simulink model "testinggrounds"  (R2022b)
settings: Solver=VariableStepAuto  StartTime=0.0  StopTime=5340  RelTol=1e-3
libraries: simulink x1, matrix_library x1
settings Model: Creator=izacu  LastModifiedBy=izacu

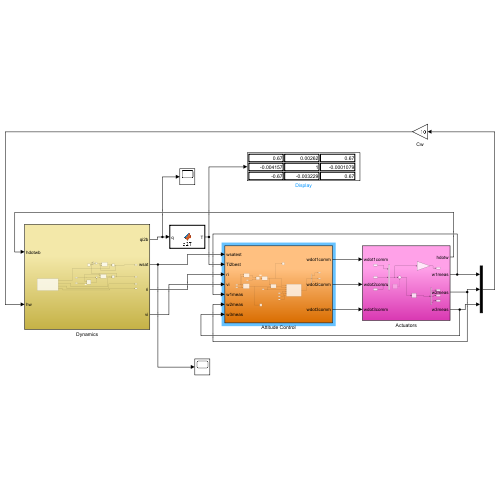
[thumbnail: Simulink's stored preview of the top-level diagram]
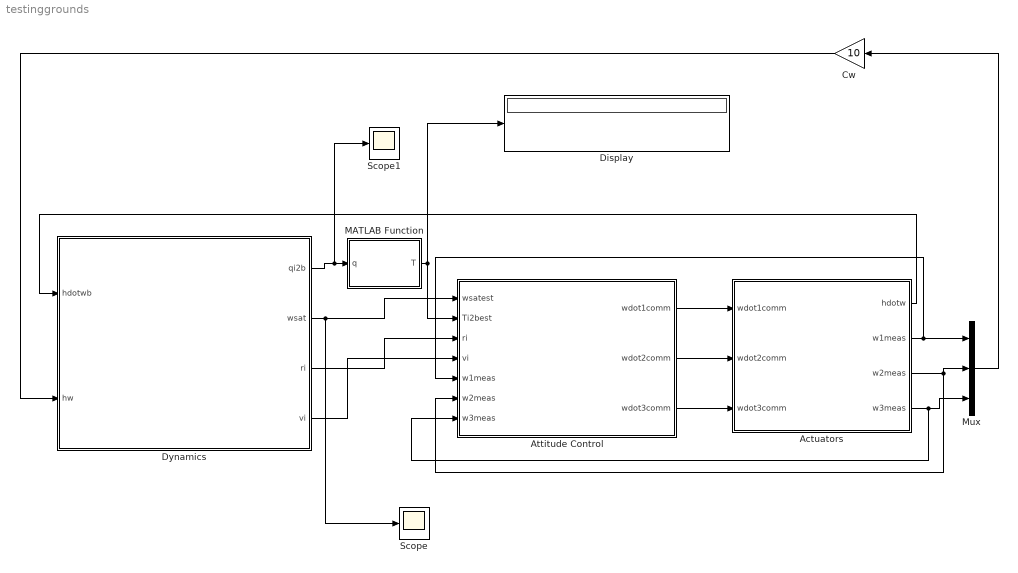
== system testinggrounds ==
  Actuators : Subsystem
  Attitude Control : Subsystem
  Cw : Gain  Gain=10
  Display : Display
  Dynamics : Subsystem
  MATLAB Function : MATLAB Function  TreatAsAtomicUnit=on
  Mux : Mux  Inputs=3
  Scope : Scope
  Scope1 : Scope
  wires:
  Attitude Control/1(wdot1comm) -> Actuators/1(wdot1comm)
  Attitude Control/2(wdot2comm) -> Actuators/2(wdot2comm)
  Attitude Control/3(wdot3comm) -> Actuators/3(wdot3comm)
  Actuators/1(hdotw) -> Dynamics/1(hdotwb)
  Actuators/2(w1meas) -> Attitude Control/5(w1meas), Mux/1
  Actuators/4(w3meas) -> Attitude Control/7(w3meas), Mux/3
  Actuators/3(w2meas) -> Mux/2, Attitude Control/6(w2meas)
  Mux/1 -> Cw/1
  Cw/1 -> Dynamics/2(hw)
  Dynamics/2(wsat) -> Scope/1, Attitude Control/1(wsatest)
  Dynamics/3(ri) -> Attitude Control/3(ri)
  Dynamics/4(vi) -> Attitude Control/4(vi)
  Dynamics/1(qi2b) -> Scope1/1, MATLAB Function/1(q)
  MATLAB Function/1(T) -> Attitude Control/2(Ti2best), Display/1

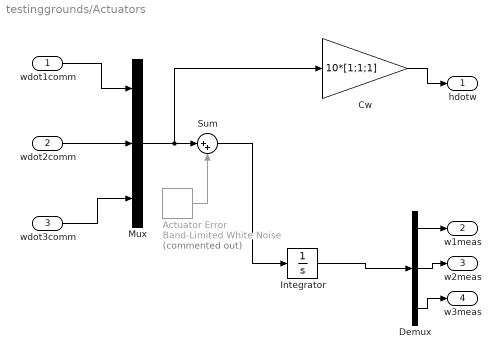
== system testinggrounds/Actuators ==
  wdot1comm : Inport
  wdot2comm : Inport  Port=2
  wdot3comm : Inport  Port=3
  Actuator Error : simulink/Sources/Band-Limited White Noise  Commented=on  Cov=1e-5 * [1;1;1]  Ts=0.1  seed=[23341]
  Cw : Gain  Gain=10*[1;1;1]
  Demux : Demux  Outputs=3
  Integrator : Integrator  InitialCondition=[0;0;0]
  Mux : Mux  Inputs=3
  Sum : Sum  Inputs=|++
  hdotw : Outport
  w1meas : Outport  Port=2
  w2meas : Outport  Port=3
  w3meas : Outport  Port=4
  wires:
  Cw/1 -> hdotw/1
  Demux/3 -> w3meas/1
  Demux/2 -> w2meas/1
  Demux/1 -> w1meas/1
  Integrator/1 -> Demux/1
  Sum/1 -> Integrator/1
  Actuator Error/1 -> Sum/2
  Mux/1 -> Sum/1, Cw/1
  wdot3comm/1 -> Mux/3
  wdot2comm/1 -> Mux/2
  wdot1comm/1 -> Mux/1

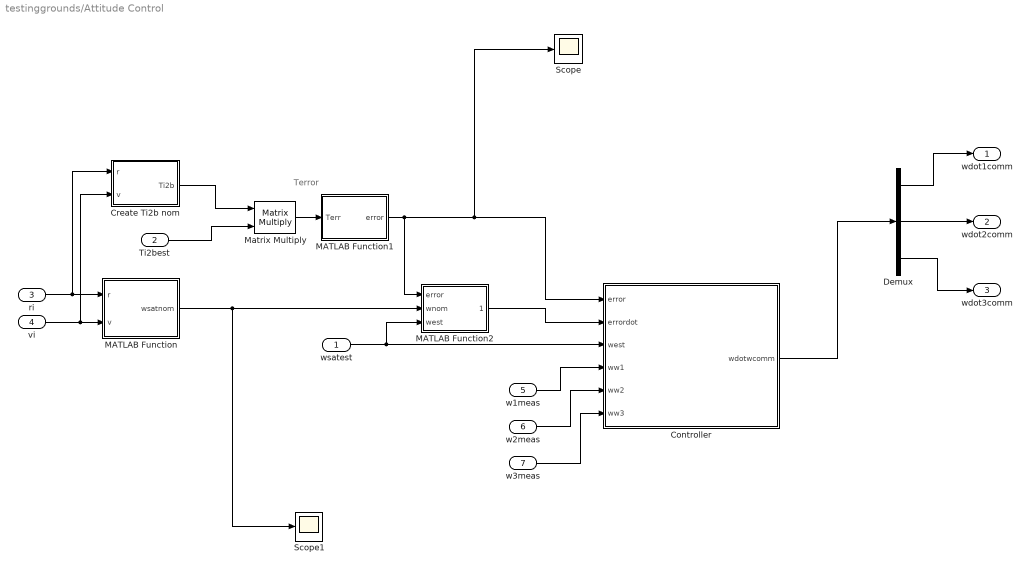
== system testinggrounds/Attitude Control ==
  note: Terror
  wsatest : Inport
  Ti2best : Inport  Port=2
  ri : Inport  Port=3
  vi : Inport  Port=4
  w1meas : Inport  Port=5
  w2meas : Inport  Port=6
  w3meas : Inport  Port=7
  Controller : MATLAB Function  TreatAsAtomicUnit=on
  Create Ti2b nom : MATLAB Function  TreatAsAtomicUnit=on
  Demux : Demux  Outputs=3
  MATLAB Function : MATLAB Function  TreatAsAtomicUnit=on
  MATLAB Function1 : MATLAB Function  TreatAsAtomicUnit=on
  MATLAB Function2 : MATLAB Function  TreatAsAtomicUnit=on
  Matrix Multiply : Product  Multiplication=Matrix(*)
  Scope : Scope
  Scope1 : Scope
  wdot1comm : Outport
  wdot2comm : Outport  Port=2
  wdot3comm : Outport  Port=3
  wires:
  MATLAB Function2/1(errordot) -> Controller/2(errordot)
  w3meas/1 -> Controller/6(ww3)
  w2meas/1 -> Controller/5(ww2)
  w1meas/1 -> Controller/4(ww1)
  wsatest/1 -> MATLAB Function2/3(west), Controller/3(west)
  MATLAB Function/1(wsatnom) -> Scope1/1, MATLAB Function2/2(wnom)
  MATLAB Function1/1(error) -> MATLAB Function2/1(error), Scope/1, Controller/1(error)
  Matrix Multiply/1 -> MATLAB Function1/1(Terr)
  vi/1 -> MATLAB Function/2(v), Create Ti2b nom/2(v)
  ri/1 -> MATLAB Function/1(r), Create Ti2b nom/1(r)
  Demux/3 -> wdot3comm/1
  Demux/2 -> wdot2comm/1
  Demux/1 -> wdot1comm/1
  Ti2best/1 -> Matrix Multiply/2
  Create Ti2b nom/1(Ti2b) -> Matrix Multiply/1
  Controller/1(wdotwcomm) -> Demux/1

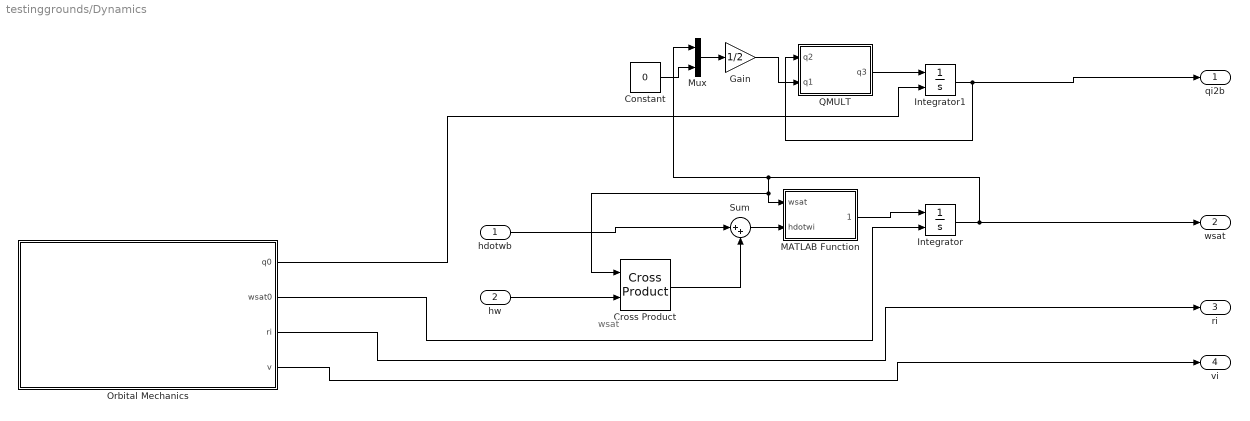
== system testinggrounds/Dynamics ==
  note: wsat
  hdotwb : Inport
  hw : Inport  Port=2
  Constant : Constant  Value=0
  Cross Product : matrix_library/Cross Product
  Gain : Gain  Gain=1/2
  Integrator : Integrator  InitialConditionSource=external
  Integrator1 : Integrator  InitialConditionSource=external
  MATLAB Function : MATLAB Function  TreatAsAtomicUnit=on
  Mux : Mux  Inputs=2
  Orbital Mechanics : Subsystem
  QMULT : MATLAB Function  TreatAsAtomicUnit=on
  Sum : Sum  Inputs=|++
  qi2b : Outport
  wsat : Outport  Port=2
  ri : Outport  Port=3
  vi : Outport  Port=4
  wires:
  Orbital Mechanics/1(q0) -> Integrator1/2
  Constant/1 -> Mux/2
  Mux/1 -> Gain/1
  QMULT/1(q3) -> Integrator1/1
  Integrator1/1 -> QMULT/1(q2), qi2b/1
  Orbital Mechanics/2(wsat0) -> Integrator/2
  Orbital Mechanics/4(v) -> vi/1
  Orbital Mechanics/3(ri) -> ri/1
  Integrator/1 -> Cross Product/1, MATLAB Function/1(wsat), Mux/1, wsat/1
  MATLAB Function/1(wdotsat) -> Integrator/1
  Sum/1 -> MATLAB Function/2(hdotwi)
  Cross Product/1 -> Sum/2
  hdotwb/1 -> Sum/1
  hw/1 -> Cross Product/2
  Gain/1 -> QMULT/2(q1)

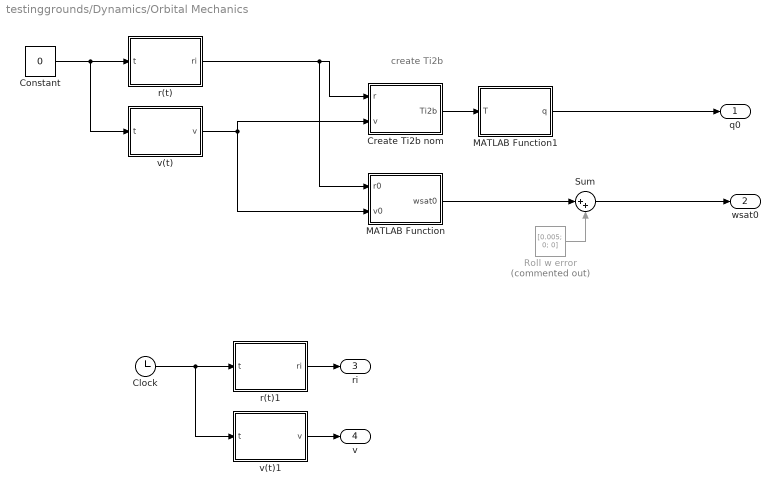
== system testinggrounds/Dynamics/Orbital Mechanics ==
  note: create Ti2b
  Clock : Clock
  Constant : Constant  Value=0
  Create Ti2b nom : MATLAB Function  TreatAsAtomicUnit=on
  MATLAB Function : MATLAB Function  TreatAsAtomicUnit=on
  MATLAB Function1 : MATLAB Function  TreatAsAtomicUnit=on
  Roll w error : Constant  Commented=on  Value=[0.005; 0; 0]
  Sum : Sum  Inputs=|++
  r(t) : MATLAB Function  TreatAsAtomicUnit=on
  r(t)1 : MATLAB Function  TreatAsAtomicUnit=on
  v(t) : MATLAB Function  TreatAsAtomicUnit=on
  v(t)1 : MATLAB Function  TreatAsAtomicUnit=on
  q0 : Outport
  wsat0 : Outport  Port=2
  ri : Outport  Port=3
  v : Outport  Port=4
  wires:
  v(t)1/1(v) -> v/1
  r(t)1/1(ri) -> ri/1
  Clock/1 -> r(t)1/1(t), v(t)1/1(t)
  MATLAB Function1/1(q) -> q0/1
  Create Ti2b nom/1(Ti2b) -> MATLAB Function1/1(T)
  Sum/1 -> wsat0/1
  MATLAB Function/1(wsat0) -> Sum/1
  Roll w error/1 -> Sum/2
  r(t)/1(ri) -> Create Ti2b nom/1(r), MATLAB Function/1(r0)
  v(t)/1(v) -> Create Ti2b nom/2(v), MATLAB Function/2(v0)
  Constant/1 -> r(t)/1(t), v(t)/1(t)

== matlab function testinggrounds/Attitude Control/Controller ==
  data: error input; wdotwcomm output; errordot input; west input; ww1 input; ww2 input; ww3 input
function wdotwcomm = fcn(error,errordot,west,ww1,ww2,ww3)
Jsat = [1000 0 0; 0 500 0; 0 0 600];
Kd = 0.05*eye(3);
Kp = 0.08*eye(3);
Cw = 10;
wdotwcomm = (Jsat*Kd ./ Cw) * error + (Jsat*Kp ./ Cw) * errordot - cross(west, [ww1; ww2; ww3]);

== matlab function testinggrounds/Dynamics/Orbital Mechanics/r(t)1 ==
  data: t input; ri output
function ri = fcn(t)

p = 6.6e6;
mu = 3.986e14;
w = sqrt(mu / (p^3));

ri = (p/sqrt(2)) * [-cos(w*t); sqrt(2)*sin(w*t); cos(w*t)];

== matlab function testinggrounds/Dynamics/MATLAB Function ==
  data: wsat input; wdotsat output; hdotwi input
function wdotsat = fcn(wsat,hdotwi)

J = [1000 0 0;
     0 500 0;
     0 0 600];

wdotsat = inv(J) * (cross(-wsat,(J*wsat)) - hdotwi); %#ok<MINV> 
end

== matlab function testinggrounds/Dynamics/Orbital Mechanics/v(t)1 ==
  data: t input; v output
function v = fcn(t)

p = 6.6e6;
mu = 3.986e14;
w = sqrt(mu / (p^3));

v = (w*p/sqrt(2)) * [sin(w*t); sqrt(2)*cos(w*t); -sin(w*t)];

== matlab function testinggrounds/Dynamics/Orbital Mechanics/r(t) ==
  data: t input; ri output
function ri = fcn(t)

p = 6.6e6;
mu = 3.986e14;
w = sqrt(mu / (p^3));

ri = (p/sqrt(2)) * [-cos(w*t); sqrt(2)*sin(w*t); cos(w*t)];

== matlab function testinggrounds/Dynamics/Orbital Mechanics/v(t) ==
  data: t input; v output
function v = fcn(t)

p = 6.6e6;
mu = 3.986e14;
w = sqrt(mu / (p^3));

v = (w*p/sqrt(2)) * [sin(w*t); sqrt(2)*cos(w*t); -sin(w*t)];

== matlab function testinggrounds/MATLAB Function ==
  data: q input; T output
function T = q2T(q)

T = eye(3) - 2*q(4)*skewsym(q(1:3)) + 2*(skewsym(q(1:3))*skewsym(q(1:3)));

end

function skewed = skewsym(v)
skewed = [0 -v(3) v(2);
          v(3) 0 -v(1);
          -v(2) v(1) 0];
end

== matlab function testinggrounds/Dynamics/QMULT ==
  data: q2 input; q3 output; q1 input
function q3 = qmult(q2,q1)

q3 = [q2(4).*q1(1:3) + q1(4).*q2(1:3) - cross(q2(1:3),q1(1:3));
    q2(4)*q1(4) - dot(q2(1:3),q1(1:3))];

end

== matlab function testinggrounds/Dynamics/Orbital Mechanics/Create Ti2b nom ==
  data: r input; Ti2b output; v input
function Ti2b = fcn(r,v)

xib = -r / norm(r);
yib = v / norm(v);
zib = cross(xib,yib);

Ti2b = [xib'; yib'; zib'];

== matlab function testinggrounds/Dynamics/Orbital Mechanics/MATLAB Function ==
  data: r0 input; wsat0 output; v0 input
function wsat0= fcn(r0,v0)
mu = 3.986e14;
rho = 6.6e6;
wmag = sqrt(mu / rho^3);

h_orbit = cross(r0,v0); % this is the axis our satellite is orbiting about
axis = h_orbit / norm(h_orbit);

wsat0 = wmag .* [0;0;1];

== matlab function testinggrounds/Dynamics/Orbital Mechanics/MATLAB Function1 ==
  data: T input; q output
function q = T2q(T)

q = zeros(4,1);

q(4) = sqrt(.25*(1 + T(1,1) + T(2,2) + T(3,3)));

q = (1/(4*q(4))) .* [T(2,3) - T(3,2); T(3,1) + T(1,3); T(1,2) + T(2,1); 4 * q(4)^2 ];

end

== matlab function testinggrounds/Attitude Control/Create Ti2b nom ==
  data: r input; Ti2b output; v input
function Ti2b = fcn(r,v)

xib = -r / norm(r);
yib = v / norm(v);
zib = cross(xib,yib);

Ti2b = [xib'; yib'; zib'];

== matlab function testinggrounds/Attitude Control/MATLAB Function ==
  data: r input; wsatnom output; v input
function wsatnom = fcn(r,v)
mu = 398600.0;
rho = 6600;
wmag = sqrt(mu / rho^3);



wsatnom = wmag .* [0;0;1];

== matlab function testinggrounds/Attitude Control/MATLAB Function1 ==
  data: Terr input; error output
function error = fcn(Terr)

error = -0.5 * [Terr(3,2) - Terr(2,3); Terr(1,3) - Terr(3,1); Terr(2,1) - Terr(1,2)];

== matlab function testinggrounds/Attitude Control/MATLAB Function2 ==
  data: error input; wnom input; errordot output; west input
function errordot = fcn(error,wnom,west)

errordot = -skewsym(wnom)*error + (-wnom + west);

end
function skewed = skewsym(v)
skewed = [0 -v(3) v(2);
          v(3) 0 -v(1);
          -v(2) v(1) 0];
end
